simulink model "MPC_Controller"  (R2023b)
settings: Solver=FixedStepAuto  StartTime=0  StopTime=10  FixedStep=0.01  RelTol=1e-3  EnableMultiTasking=on
PreLoadFcn:
  | cd extensions\simulink\pt_center_diff
  | Run_ft4wd_eclass
  | lsd_parameta_eclass
  | cd ..\..\..
InitFcn:
  | Ts = 10e-6;
  | 
  | R = 0.958;
  | Ld = 5.25e-3;
  | Lq = 12e-3;
  | Pn = 4;
  | flux = 0.1827;
  | 
  | Gi=16;
  | Gm=22;
  | Jm=0.00045;
  | Bm=0.0033;
  | Km=90;
  | mr=32;
  | Br=3620;
  | rp=0.0078
  | 
  | Tf=0.02;
  | Ff=0.2;
  | 
  | Kt=0.2
values from neighbouring files (symbols this model uses):
  lr = 1.895    [MPC_controller.m]    (also in VehicleDynamicData.m)
  m = 1270    [VehicleDynamicData.m]
  v0_ego = 20    [VehicleDynamicData.m]
  yaw0_ego = 0    [VehicleDynamicData.m]
libraries: autolibshared x1
settings Model: Creator=ywata  LastModifiedBy=aoqianzhang
settings SolverCC: AlgebraicLoopSolver=LineSearch
settings DataIOCC: SaveFormat=Array  SaveOutput=off  SaveTime=off  ReturnWorkspaceOutputs=off  SignalLoggingName=sigsOut
settings OptimizationCC: BooleanDataType=off  LifeSpan=inf
settings DebuggingCC: SaveWithParameterizedLinksMsg=none  UnderspecifiedInitializationDetection=Classic  MergeDetectMultiDrivingBlocksExec=none  SignalResolutionControl=TryResolveAllWithWarning  MultiTaskDSMMsg=warning  MultiTaskCondExecSysMsg=none  FcnCallInpInsideContextMsg=warning  UnconnectedInputMsg=warning  UnconnectedOutputMsg=warning  UnconnectedLineMsg=warning  StateNameClashWarn=warning  SFUnexpectedBacktrackingDiag=warning  SFNoUnconditionalDefaultTransitionDiag=warning  SFExecutionAtInitializationDiag=none  ArithmeticOperatorsInVariantConditions=warning
settings HardwareCC: ProdBitPerPointer=32  ProdBitPerSizeT=32  ProdBitPerPtrDiffT=32  ProdLargestAtomicFloat=None  ProdIntDivRoundTo=Undefined  ProdEndianess=Unspecified  ProdWordSize=32  ProdHWDeviceType=32-bit Generic  TargetBitPerLong=64  TargetBitPerPointer=64  TargetBitPerSizeT=64  TargetBitPerPtrDiffT=64  TargetLongLongMode=on  TargetIntDivRoundTo=Zero  TargetEndianess=LittleEndian  TargetWordSize=64  TargetHWDeviceType=MATLAB Host  ProdEqTarget=off
settings ModelReferenceCC: EnableRefExpFcnMdlSchedulingChecks=on  PropagateSignalLabelsOutOfModel=off
settings SFSimCC: SimUseLocalCustomCode=off  CustomCodeUndefinedFunction=UseInterfaceOnly
settings RTWCC: RTWUseLocalCustomCode=off  DLArmComputeVersion=19.05
settings CodeAppCC: StateflowObjectComments=on
settings GRTTargetCC: TargetFcnLib=ansi_tfl_tmw.mat  TargetLangStandard=C89/C90 (ANSI)  ModelReferenceCompliant=off  CombineOutputUpdateFcns=off  MatFileLogging=off  GRTInterface=on
settings ConfigComp: CovMetricSettings=dw  CovSaveCumulativeToWorkspaceVar=on  CovSaveSingleToWorkspaceVar=on  CovExternalEMLEnable=off

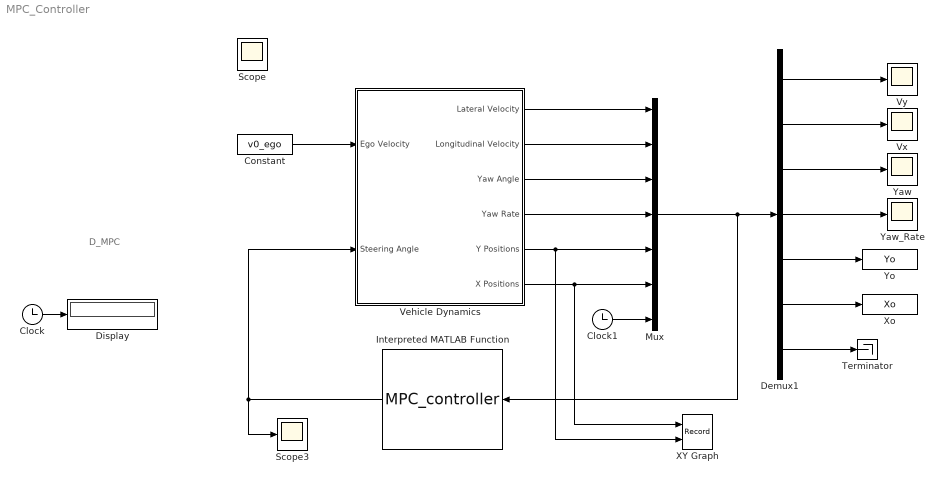
== system MPC_Controller ==
  note: D_MPC
  Clock : Clock
  Clock1 : Clock
  Constant : Constant  Value=v0_ego
  Demux1 : Demux  Outputs=7
      settings: DisplayOption=none
  Display : Display
  Interpreted MATLAB Function : MATLABFcn  MATLABFcn=MPC_controller  OutputDimensions=1  Output1D=off
  Mux : Mux  Inputs=7
  Scope3 : Scope
  Terminator : Terminator
  Vehicle Dynamics : Subsystem  VariantControl=VariantVDBS
  Vx : Scope
  Vy : Scope
  XY Graph : Record  FileSettingsInternal="{\"entries\":[{\"content\":{\"excelSettings\":{\"content\":{},\"type\":\"Streamout.ExcelSettings\"}},\"type\":\"Streamout.FileSettingStorage\",\"uuid\":\"\"}],\"packageUris\":[\"http:\\/\\/schema.mathworks.com\\/mf0\\/streamout_blocks\\/R2020a\"],\"version\":\"1.0\"}"  Layout=[1 1]  SignalsInternal="{\"entries\":[{\"content\":{\"signals\":[{\"content\":{\"blockPath\":[],\"dimensions\":[1],\"domain\":\"\",\"lineColor\":\"#a2142f\",\"plots\":[1],\"port\":1,\"signalID\":732,\"signalName\":\"Vehicle Dynamics:6\"},\"type\":\"RecordBlkView.Signal\",\"uuid\":\"\"},{\"content\":{\"blockPath\":[],\"dimensions\":[1],\"domain\":\"\",\"lineColor\":\"#139fff\",\"plots\":[1],\"port\":2,\"signalID\":735,\"signalName\":\"Vehicle Dynamics:5\"},\"type\":\"RecordBlkView.Signal\",\"uuid\":\"\"}]},\"type\":\"RecordBlkView.InputSignals\",\"uuid\":\"\"}],\"packageUris\":[\"http:\\/\\/schema.mathworks.com\\/mf0\\/streamout_blocks\\/R2020a\"],\"version\":\"1.0\"}"  VisualizationBindings="{\"xyplotplugin\":{\"info\":[{\"series\":[{\"bindingParametersList\":[{\"parameter\":\"X-Axis\",\"signalID\":732,\"signalName\":\"Vehicle Dynamics:6\"},{\"parameter\":\"Y-Axis\",\"signalID\":735,\"signalName\":\"Vehicle Dynamics:5\"}],\"seriesID\":48619}],\"subplotID\":1}]}}"  CompatibilityTag=XY  st=-1
  Xo : ToWorkspace  VariableName=Xo  SaveFormat=Structure With Time  SampleTime=-1
  Yaw : Scope
  Yaw_Rate : Scope
  Yo : ToWorkspace  VariableName=Yo  SaveFormat=Structure With Time  SampleTime=-1
  Scope : Scope
  wires:
  Clock/1 -> Display/1
  Demux1/4 -> Yaw_Rate/1
  Demux1/3 -> Yaw/1
  Demux1/2 -> Vx/1
  Demux1/1 -> Vy/1
  Mux/1 -> Demux1/1, Interpreted MATLAB Function/1
  Demux1/5 -> Yo/1
  Demux1/6 -> Xo/1
  Constant/1 -> Vehicle Dynamics/1(Ego Velocity)
  Interpreted MATLAB Function/1 -> Vehicle Dynamics/2(Steering Angle), Scope3/1
  Vehicle Dynamics/1(Lateral Velocity) -> Mux/1
  Vehicle Dynamics/2(Longitudinal Velocity) -> Mux/2
  Vehicle Dynamics/3(Yaw Angle) -> Mux/3
  Vehicle Dynamics/4(Yaw Rate) -> Mux/4
  Vehicle Dynamics/5(Y Positions) -> Mux/5, XY Graph/2
  Vehicle Dynamics/6(X Positions) -> Mux/6, XY Graph/1
  Clock1/1 -> Mux/7
  Demux1/7 -> Terminator/1

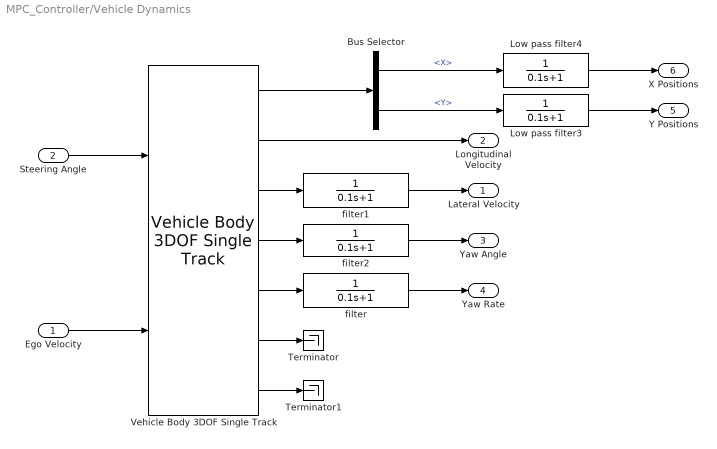
== system MPC_Controller/Vehicle Dynamics ==
  Ego Velocity : Inport
  Steering Angle : Inport  Port=2
  Bus Selector : BusSelector  OutputSignals=InertFrm.Cg.Disp.X,InertFrm.Cg.Disp.Y
  Low pass filter3 : TransferFcn  Denominator=[0.1 1]
  Low pass filter4 : TransferFcn  Denominator=[0.1 1]
  Terminator : Terminator
  Terminator1 : Terminator
  Vehicle Body 3DOF Single Track : autolibshared/Vehicle Body 3DOF Single Track  trackMode=Single (bicycle)  inputMode=External longitudinal velocity  frontSteerMode=on  rearSteerMode=off  windMode=off  muMode=off  extFMode=off  extMMode=off  htchFMode=off  htchMMode=off  extXo=off  extpsio=off  extxdoto=off  extro=off  extYo=off  extTamb=off  extydoto=off  aMode=2  NF=2  NR=2  m=m  a=lf  b=lr  h=0.35  dh=1  hh=0.2  X_o=x0_ego  xdot_o=0  CalphaMode=off  sigmaMode=on  d=0  hl=0  w=[1.4,1.4]  Cy_f=Cf  Cy_r=Cr  sigma_f=.1  sigma_r=.1  alpha_f_brk=[-.1 .1]  Cy_f_data=[-9e3 9e3]  alpha_r_brk=[-.1 .1]  Cy_r_data=[-9e3 9e3]  Y_o=y0_ego  ydot_o=0  Izz=Iz  psi_o=yaw0_ego*pi/180  r_o=0  Af=0  Cd=.3  Cl=.1  Cpm=.1  beta_w=[0:0.01:0.3]  Cs=[0:0.03:0.9]  Cym=[0:0.01:0.3]  Pabs=101325  Tair=273  g=9.81  mu=1  xdot_tol=.01  Fznom=m*9.81  Fxtire_sat=7e4  Fytire_sat=7e4  longOff=0  latOff=0  vertOff=0  wrapAng=off
  filter : TransferFcn  Denominator=[0.1 1]
  filter1 : TransferFcn  Denominator=[0.1 1]
  filter2 : TransferFcn  Denominator=[0.1 1]
  Lateral Velocity : Outport  Unit=m/s  VectorParamsAs1DForOutWhenUnconnected=off
  Longitudinal Velocity : Outport  Port=2  Unit=m/s  VectorParamsAs1DForOutWhenUnconnected=off
  Yaw Angle : Outport  Port=3  Unit=deg  VectorParamsAs1DForOutWhenUnconnected=off
  Yaw Rate : Outport  Port=4  Unit=degree/s  VectorParamsAs1DForOutWhenUnconnected=off
  Y Positions : Outport  Port=5  Unit=m  VectorParamsAs1DForOutWhenUnconnected=off
  X Positions : Outport  Port=6  Unit=m  VectorParamsAs1DForOutWhenUnconnected=off
  wires:
  Ego Velocity/1 -> Vehicle Body 3DOF Single Track/2
  Vehicle Body 3DOF Single Track/1 -> Bus Selector/1
  Vehicle Body 3DOF Single Track/2 -> Longitudinal Velocity/1
  Bus Selector/1 -> Low pass filter4/1  "<X>"
  Bus Selector/2 -> Low pass filter3/1  "<Y>"
  Vehicle Body 3DOF Single Track/5 -> filter/1
  Steering Angle/1 -> Vehicle Body 3DOF Single Track/1
  filter/1 -> Yaw Rate/1
  Vehicle Body 3DOF Single Track/3 -> filter1/1
  filter1/1 -> Lateral Velocity/1
  filter2/1 -> Yaw Angle/1
  Vehicle Body 3DOF Single Track/4 -> filter2/1
  Low pass filter3/1 -> Y Positions/1
  Low pass filter4/1 -> X Positions/1
  Vehicle Body 3DOF Single Track/6 -> Terminator/1
  Vehicle Body 3DOF Single Track/7 -> Terminator1/1
